simulink model "APPS_Simulation"  (R2024a)
settings: Solver=FixedStepDiscrete  StartTime=0.0  StopTime=10  FixedStep=0.001  RelTol=1e-3
libraries: simulink x4
settings Model: Creator=laszlokilyen  LastModifiedBy=laszlokilyen

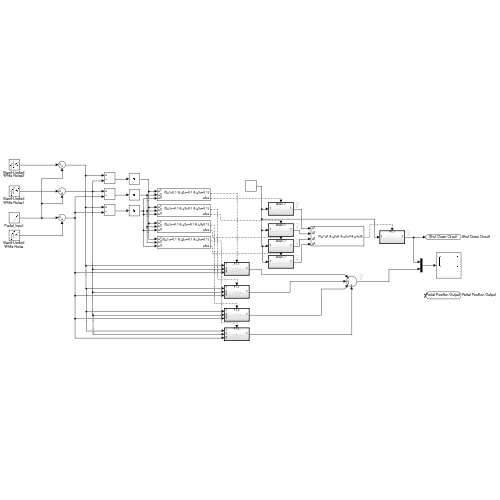
[thumbnail: Simulink's stored preview of the top-level diagram]
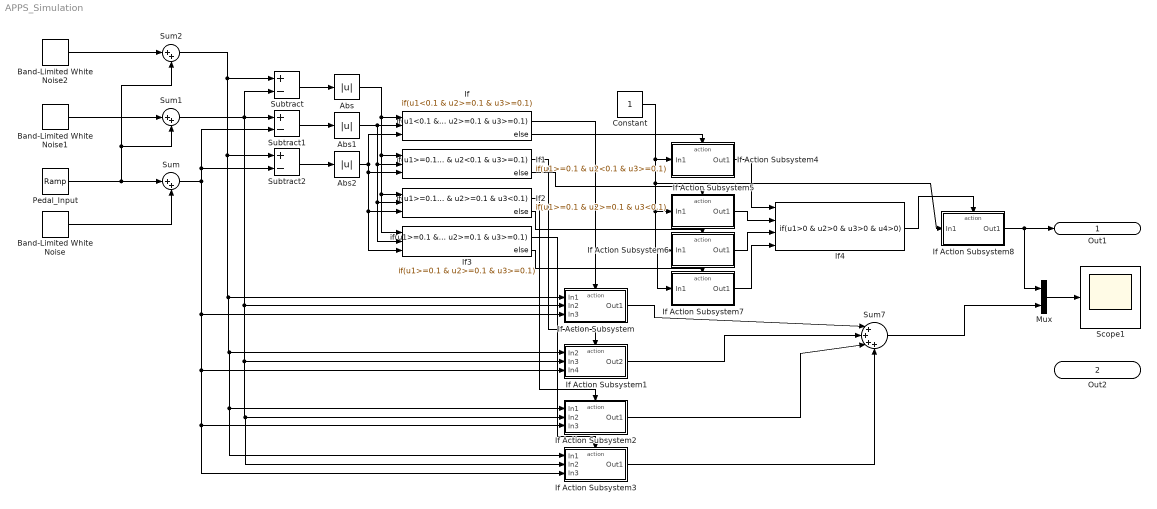
== system APPS_Simulation ==
  Abs : Abs  SaturateOnIntegerOverflow=off
  Abs1 : Abs  SaturateOnIntegerOverflow=off
  Abs2 : Abs  SaturateOnIntegerOverflow=off
  Band-Limited White Noise : simulink/Sources/Band-Limited White Noise  Cov=[0.00001]  Ts=0.1  seed=[23341]
  Band-Limited White Noise1 : simulink/Sources/Band-Limited White Noise  Cov=[0.001]  Ts=0.1  seed=[23341]
  Band-Limited White Noise2 : simulink/Sources/Band-Limited White Noise  Cov=[0.001]  Ts=0.1  seed=[23341]
  Constant : Constant
  If : If  NumInputs=3  IfExpression=u1<0.1 & u2>=0.1 & u3>=0.1
  If Action Subsystem : Subsystem  TreatAsAtomicUnit=on
  If Action Subsystem1 : Subsystem  TreatAsAtomicUnit=on
  If Action Subsystem2 : Subsystem  TreatAsAtomicUnit=on
  If Action Subsystem3 : Subsystem  TreatAsAtomicUnit=on
  If Action Subsystem4 : Subsystem  TreatAsAtomicUnit=on
  If Action Subsystem5 : Subsystem  TreatAsAtomicUnit=on
  If Action Subsystem6 : Subsystem  TreatAsAtomicUnit=on
  If Action Subsystem7 : Subsystem  TreatAsAtomicUnit=on
  If Action Subsystem8 : Subsystem  TreatAsAtomicUnit=on
  If1 : If  NumInputs=3  IfExpression=u1>=0.1 & u2<0.1 & u3>=0.1
  If2 : If  NumInputs=3  IfExpression=u1>=0.1 & u2>=0.1 & u3<0.1
  If3 : If  NumInputs=3  IfExpression=u1>=0.1 & u2>=0.1 & u3>=0.1
  If4 : If  NumInputs=4  IfExpression=u1>0 & u2>0 & u3>0 & u4>0  ShowElse=off
  Mux : Mux  Inputs=2
  Pedal_Input : simulink/Sources/Ramp  slope=10  start=0  InitialOutput=0
  Scope1 : Scope
  Subtract : Sum  Inputs=+-
  Subtract1 : Sum  Inputs=+-
  Subtract2 : Sum  Inputs=+-
  Sum : Sum  Inputs=|++
  Sum1 : Sum  Inputs=|++
  Sum2 : Sum  Inputs=|++
  Sum7 : Sum  Inputs=|++++
  Out1 : Outport  SignalName=Shut Down Circuit
  Out2 : Outport  Port=2  SignalName=Pedal Position Output
  wires:
  Band-Limited White Noise/1 -> Sum/2
  Band-Limited White Noise1/1 -> Sum1/1
  Band-Limited White Noise2/1 -> Sum2/1
  Pedal_Input/1 -> Sum/1, Sum2/2, Sum1/2
  Subtract/1 -> Abs/1
  Subtract1/1 -> Abs1/1
  Subtract2/1 -> Abs2/1
  Sum/1 -> If Action Subsystem3/3(In3), If Action Subsystem2/3(In3), If Action Subsystem1/3(In4), If Action Subsystem/3(In3), Subtract1/2, Subtract2/2
  Sum2/1 -> If Action Subsystem3/1(In1), If Action Subsystem2/1(In1), If Action Subsystem1/1(In2), If Action Subsystem/1(In1), Subtract2/1, Subtract/1
  Abs/1 -> If3/1, If2/1, If1/1, If/1
  Abs1/1 -> If3/2, If2/2, If1/2, If/2
  Abs2/1 -> If/3, If3/3, If2/3, If1/3
  If/2 -> If Action Subsystem4/Action
  If1/2 -> If Action Subsystem5/Action
  If2/2 -> If Action Subsystem6/Action
  If3/2 -> If Action Subsystem7/Action
  If/1 -> If Action Subsystem/Action
  If1/1 -> If Action Subsystem1/Action
  If2/1 -> If Action Subsystem2/Action
  If3/1 -> If Action Subsystem3/Action
  If Action Subsystem/1(Out1) -> Sum7/1
  If Action Subsystem1/1(Out2) -> Sum7/2
  If Action Subsystem2/1(Out1) -> Sum7/3
  If Action Subsystem3/1(Out1) -> Sum7/4
  Sum1/1 -> If Action Subsystem3/2(In2), If Action Subsystem2/2(In2), If Action Subsystem1/2(In3), If Action Subsystem/2(In2), Subtract/2, Subtract1/1
  Constant/1 -> If Action Subsystem8/1(In1), If Action Subsystem7/1(In1), If Action Subsystem6/1(In1), If Action Subsystem5/1(In1), If Action Subsystem4/1(In1)
  If Action Subsystem4/1(Out1) -> If4/1
  If Action Subsystem5/1(Out1) -> If4/2
  If Action Subsystem6/1(Out1) -> If4/3
  If Action Subsystem7/1(Out1) -> If4/4
  If4/1 -> If Action Subsystem8/Action
  If Action Subsystem8/1(Out1) -> Mux/1, Out1/1
  Mux/1 -> Scope1/1
  Sum7/1 -> Mux/2

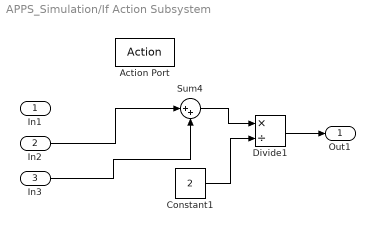
== system APPS_Simulation/If Action Subsystem ==
  In1 : Inport
  In2 : Inport  Port=2
  In3 : Inport  Port=3
  Action Port : ActionPort  ActionPortLabel=if(u1<0.1 & u2>=0.1 & u3>=0.1)
  Constant1 : Constant  Value=2
  Divide1 : Product  Inputs=*/
  Sum4 : Sum  Inputs=|++
  Out1 : Outport
  wires:
  Divide1/1 -> Out1/1
  Constant1/1 -> Divide1/2
  Sum4/1 -> Divide1/1
  In3/1 -> Sum4/2
  In2/1 -> Sum4/1

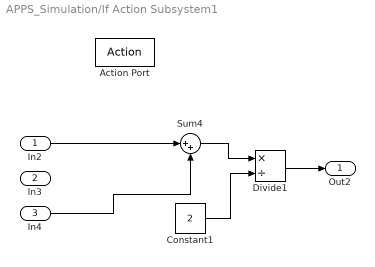
== system APPS_Simulation/If Action Subsystem1 ==
  In2 : Inport
  In3 : Inport  Port=2
  In4 : Inport  Port=3
  Action Port : ActionPort  ActionPortLabel=if(u1>=0.1 & u2<0.1 & u3>=0.1)
  Constant1 : Constant  Value=2
  Divide1 : Product  Inputs=*/
  Sum4 : Sum  Inputs=|++
  Out2 : Outport
  wires:
  In4/1 -> Sum4/2
  Sum4/1 -> Divide1/1
  Constant1/1 -> Divide1/2
  Divide1/1 -> Out2/1
  In2/1 -> Sum4/1

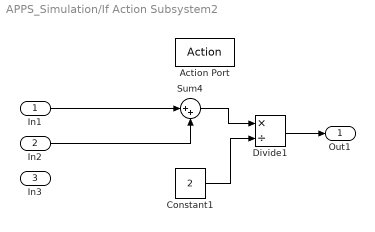
== system APPS_Simulation/If Action Subsystem2 ==
  In1 : Inport
  In2 : Inport  Port=2
  In3 : Inport  Port=3
  Action Port : ActionPort  ActionPortLabel=if(u1>=0.1 & u2>=0.1 & u3<0.1)
  Constant1 : Constant  Value=2
  Divide1 : Product  Inputs=*/
  Sum4 : Sum  Inputs=|++
  Out1 : Outport
  wires:
  Sum4/1 -> Divide1/1
  Constant1/1 -> Divide1/2
  Divide1/1 -> Out1/1
  In1/1 -> Sum4/1
  In2/1 -> Sum4/2

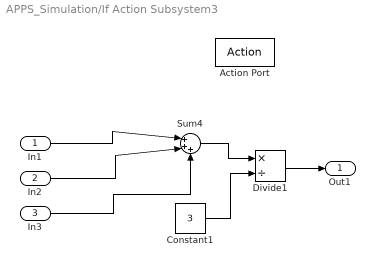
== system APPS_Simulation/If Action Subsystem3 ==
  In1 : Inport
  In2 : Inport  Port=2
  In3 : Inport  Port=3
  Action Port : ActionPort  ActionPortLabel=if(u1>=0.1 & u2>=0.1 & u3>=0.1)
  Constant1 : Constant  Value=3
  Divide1 : Product  Inputs=*/
  Sum4 : Sum  Inputs=|+++
  Out1 : Outport
  wires:
  Sum4/1 -> Divide1/1
  Constant1/1 -> Divide1/2
  Divide1/1 -> Out1/1
  In1/1 -> Sum4/1
  In2/1 -> Sum4/2
  In3/1 -> Sum4/3

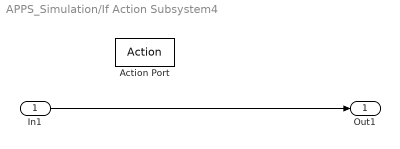
== system APPS_Simulation/If Action Subsystem4 ==
  In1 : Inport
  Action Port : ActionPort  ActionPortLabel=else
  Out1 : Outport
  wires:
  In1/1 -> Out1/1

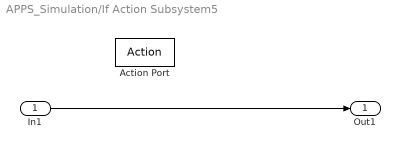
== system APPS_Simulation/If Action Subsystem5 ==
  In1 : Inport
  Action Port : ActionPort  ActionPortLabel=else
  Out1 : Outport
  wires:
  In1/1 -> Out1/1

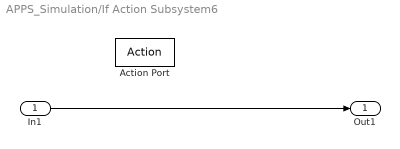
== system APPS_Simulation/If Action Subsystem6 ==
  In1 : Inport
  Action Port : ActionPort  ActionPortLabel=else
  Out1 : Outport
  wires:
  In1/1 -> Out1/1

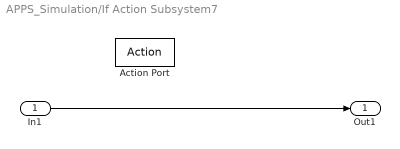
== system APPS_Simulation/If Action Subsystem7 ==
  In1 : Inport
  Action Port : ActionPort  ActionPortLabel=else
  Out1 : Outport
  wires:
  In1/1 -> Out1/1

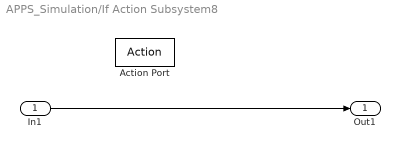
== system APPS_Simulation/If Action Subsystem8 ==
  In1 : Inport
  Action Port : ActionPort  ActionPortLabel=if(u1>0 & u2>0 & u3>0 & u4>0)
  Out1 : Outport
  wires:
  In1/1 -> Out1/1
